simulink model "dyanmics_model"  (R2018b)
settings: Solver=VariableStepAuto  StartTime=0.0  StopTime=100.0  RelTol=1e-3
values from neighbouring files (symbols this model uses):
  aeroCoeff =     [flight_params.mat]
  alpha = [-15 -14 -13 -12 -11 -10 -9 -8 -7 -6 -5 -4 ... (31 elements, 1x31)]    [flight_params.mat]
  cjet = [0 1 2 3 4 5 6 7 8 9 10 11 ... (21 elements, 1x21)]    [flight_params.mat]
  CLtot = [-1.4145 -1.8537 -2.1722 -2.4757 -2.7723 -3.0649 -3.3548 -3.6428 -3.9294 -4.215 -4.4997 -4.7837 ... (13325 elements, 13x25x41)]    [flight_params.mat]
  CXtot = [0.3779 0.8471 1.6222 2.448 3.3002 4.1691 5.0501 5.94 6.8372 7.7403 8.6483 9.5605 ... (13325 elements, 13x25x41)]    [flight_params.mat]
  CZtot = [1.3677 1.6644 1.7212 1.7436 1.749 1.7441 1.732 1.7146 1.6931 1.6682 1.6407 1.6109 ... (13325 elements, 13x25x41)]    [flight_params.mat]
  environment =     [flight_params.mat]
  flap = [-10 -5 0 5 10 15 20 25 30 35 40 45 ... (21 elements, 1x21)]    [flight_params.mat]
  InitialConditions =     [flight_params.mat]
  vehicle =     [flight_params.mat]
libraries: simulink_extras x5, aerolibasang x2, shared3dof x1, sharedtransform x1
settings Model: Creator=Jacob  LastModifiedBy=Jacob

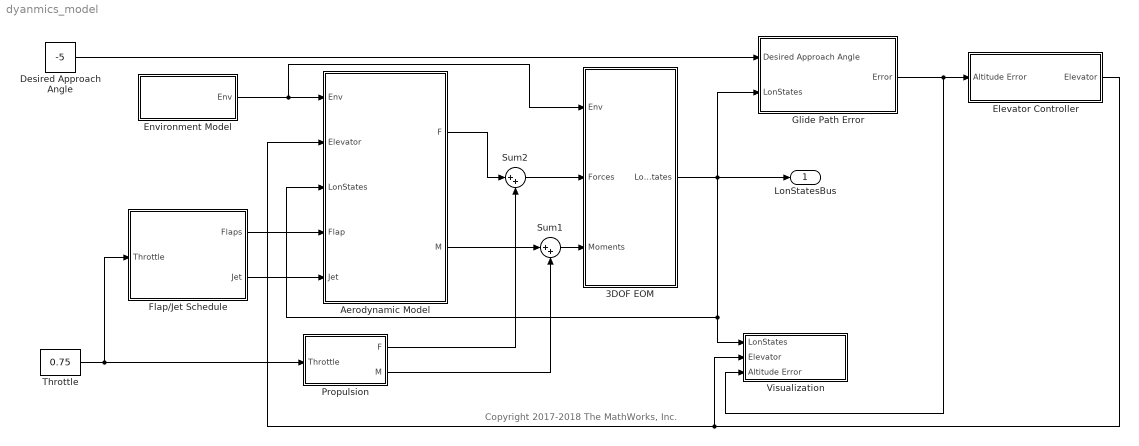
== system dyanmics_model ==
  note: Copyright 2017-2018 The MathWorks, Inc.
  3DOF EOM : Subsystem  VariantControl=eom3DOF
  Aerodynamic Model : Subsystem  VariantControl=aeroCONST
  Desired Approach Angle : Constant  Value=-5
  Elevator Controller : Subsystem
  Environment Model : Subsystem  mask(Constant Environment Model){To=environment.T0, a=environment.a, Po=environment.P0, AirDensity=environment.rho0, ugvgwg=environment.vel_wind, pgqgrg=environment.omega_wind, g=environment.grav}
      mask prompts: To "Constant Temperature (K):"; a "Constant Speed of Sound (m/s):"; Po "Constant Pressure (Pa):"; AirDensity "Constant Air Density (kg/m^3):"; ugvgwg "Constant Wind Velocity [ug vg wg] (m/s):"; pgqgrg "Constant Wind Angular Rates [pg qg rg] (rad/s):"; g "Constant Gravitational Acceleration (m/s^2):"
      mask Help: helpview(fullfile(docroot,'toolbox','aeroblks','aeroblks.map'), 'environment1');
      mask TypeOptions To: Constant Atmosphere/To
      mask TypeOptions a: Constant Atmosphere/a
      mask TypeOptions Po: Constant Atmosphere/Po
      mask TypeOptions AirDensity: Constant Atmosphere/AirDensity
      mask TypeOptions ugvgwg: Constant Wind/ugvgwg
      mask TypeOptions pgqgrg: Constant Wind/pgqgrg
      mask TypeOptions g: Constant Gravity/g
      mask DialogControl Container4 Prompt: Atmospheric Model
      mask DialogControl Container6 Prompt: Wind Model
      mask DialogControl Container8 Prompt: Gravity Model
      mask Display:
      | image('aeroenvironment.bmp','center')
      | port_label('output',1,'Env')
  Flap/Jet Schedule : Subsystem
  Glide Path Error : Subsystem
  Propulsion : Subsystem
      settings: RTWSystemCode=Inline
  Sum1 : Sum  Inputs=|++  SaturateOnIntegerOverflow=on  InputSameDT=on  OutDataTypeStr=Inherit: Same as first input
  Sum2 : Sum  Inputs=|++  SaturateOnIntegerOverflow=on  InputSameDT=on  OutDataTypeStr=Inherit: Same as first input
  Throttle : Constant  Value=0.75
  Visualization : Subsystem
  LonStatesBus : Outport
  wires:
  Propulsion/2(M) -> Sum1/2
  Propulsion/1(F) -> Sum2/2
  Environment Model/1(Env) -> 3DOF EOM/1(Env), Aerodynamic Model/1(Env)
  Sum1/1 -> 3DOF EOM/3(Moments)
  Aerodynamic Model/1(F) -> Sum2/1
  3DOF EOM/1(LonStates) -> Visualization/1(LonStates), Aerodynamic Model/3(LonStates), LonStatesBus/1, Glide Path Error/2(LonStates)
  Throttle/1 -> Flap/Jet Schedule/1(Throttle), Propulsion/1(Throttle)
  Sum2/1 -> 3DOF EOM/2(Forces)
  Aerodynamic Model/2(" M") -> Sum1/1
  Flap/Jet Schedule/2(Jet) -> Aerodynamic Model/5(Jet)
  Flap/Jet Schedule/1(Flaps) -> Aerodynamic Model/4(Flap)
  Desired Approach Angle/1 -> Glide Path Error/1(Desired Approach Angle)
  Glide Path Error/1(Error) -> Elevator Controller/1(Altitude Error), Visualization/3(Altitude Error)
  Elevator Controller/1(Elevator) -> Visualization/2(Elevator), Aerodynamic Model/2(Elevator)

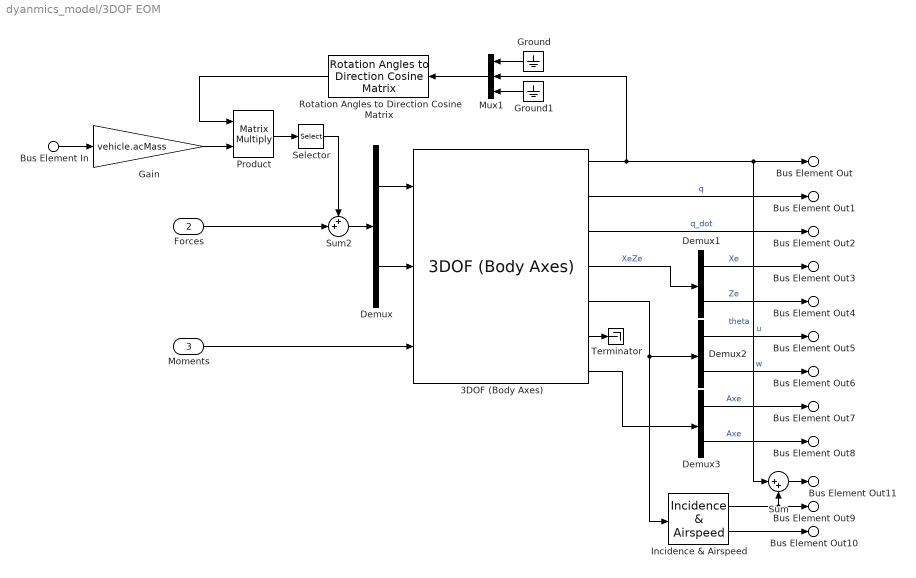
== system dyanmics_model/3DOF EOM ==
  Bus Element In : Inport  PortName=Env  Element=g
  Forces : Inport  Port=2
  Moments : Inport  Port=3
  3DOF (Body Axes) : shared3dof/3DOF (Body Axes)  units=Metric (MKS)  mtype=Fixed  v_ini=InitialConditions.v0  theta_ini=InitialConditions.theta0  alpha_ini=InitialConditions.alpha0  pos_ini=InitialConditions.x0  q_ini=InitialConditions.q0  mass=vehicle.acMass  mass_e=0.5  mass_f=3.0  Iyy=vehicle.inertia_yy  Iyy_e=0.5  Iyy_f=3.0  g_in=Internal  g=0  vre_flag=on  abi_flag=on  aMode=0  vel_statename={'u', 'w'}  theta_statename='theta'  pos_statename={'Xe', 'Ze'}  q_statename='q'  mass_statename=''
      settings: SourceProductName=Aerospace Blockset  SourceProductBaseCode=AE
  Demux{,1..3} (4 alike) : Demux  Outputs=2
  Gain : Gain  Gain=vehicle.acMass
  Ground : Ground
  Ground1 : Ground
  Incidence & Airspeed : aerolibasang/Incidence  & Airspeed
      settings: SourceProductName=Aerospace Blockset  SourceProductBaseCode=AE
  Mux1 : Mux  Inputs=3
  Product : Product  Multiplication=Matrix(*)
  Rotation Angles to Direction Cosine Matrix : sharedtransform/Rotation Angles to Direction Cosine Matrix  rotationOrder=ZYX  aMode=aMode
      settings: SourceProductBaseCode=AE
  Selector : Selector  InputPortWidth=3  IndexOptions=Index vector (dialog)  Indices=[1 3]  OutputSizes=1
  Sum : Sum  Inputs=|++
  Sum2 : Sum  Inputs=++|  SaturateOnIntegerOverflow=on  InputSameDT=on  OutDataTypeStr=Inherit: Same as first input
  Terminator : Terminator
  Bus Element Out : Outport  PortName=LonStates  Element=theta
  Bus Element Out1 : Outport  PortName=LonStates  Element=q
  Bus Element Out2 : Outport  PortName=LonStates  Element=q_dot
  Bus Element Out3 : Outport  PortName=LonStates  Element=Xe
  Bus Element Out4 : Outport  PortName=LonStates  Element=Ze
  Bus Element Out5 : Outport  PortName=LonStates  Element=u
  Bus Element Out6 : Outport  PortName=LonStates  Element=w
  Bus Element Out7 : Outport  PortName=LonStates  Element=Axe
  Bus Element Out8 : Outport  PortName=LonStates  Element=Aze
  Bus Element Out9 : Outport  PortName=LonStates  Element=alpha
  Bus Element Out10 : Outport  PortName=LonStates  Element=v
  Bus Element Out11 : Outport  PortName=LonStates  Element=gamma
  wires:
  Demux/2 -> 3DOF (Body Axes)/2
  Demux/1 -> 3DOF (Body Axes)/1
  Sum2/1 -> Demux/1
  Selector/1 -> Sum2/1
  Ground1/1 -> Mux1/3
  Ground/1 -> Mux1/1
  Mux1/1 -> Rotation Angles to Direction Cosine Matrix/1
  Gain/1 -> Product/2
  Rotation Angles to Direction Cosine Matrix/1 -> Product/1
  Product/1 -> Selector/1
  Forces/1 -> Sum2/2
  Bus Element In/1 -> Gain/1
  Moments/1 -> 3DOF (Body Axes)/3
  3DOF (Body Axes)/1 -> Mux1/2, Bus Element Out/1, Sum/1  "theta"
  3DOF (Body Axes)/2 -> Bus Element Out1/1  "q"
  3DOF (Body Axes)/3 -> Bus Element Out2/1  "q_dot"
  3DOF (Body Axes)/4 -> Demux1/1  "XeZe"
  3DOF (Body Axes)/5 -> Incidence & Airspeed/1, Demux2/1
  3DOF (Body Axes)/7 -> Demux3/1
  Demux3/1 -> Bus Element Out7/1  "Axe"
  Demux3/2 -> Bus Element Out8/1  "Axe"
  Demux2/2 -> Bus Element Out6/1  "w"
  Demux2/1 -> Bus Element Out5/1  "u"
  Demux1/2 -> Bus Element Out4/1  "Ze"
  Demux1/1 -> Bus Element Out3/1  "Xe"
  3DOF (Body Axes)/6 -> Terminator/1
  Incidence & Airspeed/1 -> Bus Element Out9/1, Sum/2
  Incidence & Airspeed/2 -> Bus Element Out10/1
  Sum/1 -> Bus Element Out11/1

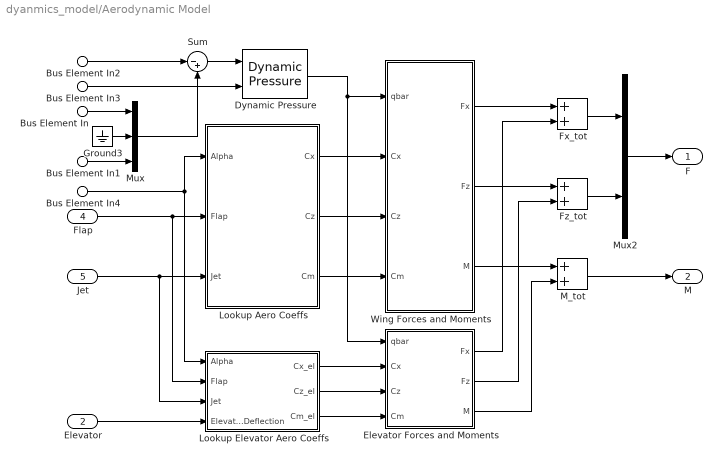
== system dyanmics_model/Aerodynamic Model ==
  Bus Element In2 : Inport  PortName=Env  Element=WindVelocity
  Bus Element In3 : Inport  PortName=Env  Element=AirDensity
  Elevator : Inport  Port=2
  Bus Element In : Inport  Port=3  PortName=LonStates  Element=u
  Bus Element In1 : Inport  Port=3  PortName=LonStates  Element=w
  Bus Element In4 : Inport  Port=3  PortName=LonStates  Element=alpha
  Flap : Inport  Port=4
  Jet : Inport  Port=5
  Dynamic Pressure : aerolibasang/Dynamic Pressure
  Elevator Forces and Moments : Subsystem
  Fx_tot : Sum  SaturateOnIntegerOverflow=on  InputSameDT=on  OutDataTypeStr=Inherit: Same as first input
  Fz_tot : Sum  SaturateOnIntegerOverflow=on  InputSameDT=on  OutDataTypeStr=Inherit: Same as first input
  Ground3 : Ground
  Lookup Aero Coeffs : Subsystem
  Lookup Elevator Aero Coeffs : Subsystem
  M_tot : Sum  SaturateOnIntegerOverflow=on  InputSameDT=on  OutDataTypeStr=Inherit: Same as first input
  Mux : Mux  Inputs=3
  Mux2 : Mux  Inputs=2
  Sum : Sum  Inputs=|-+
  Wing Forces and Moments : Subsystem
  F : Outport
  " M" : Outport  Port=2  Unit=N*m
  wires:
  Bus Element In3/1 -> Dynamic Pressure/2
  Bus Element In2/1 -> Sum/1
  Bus Element In/1 -> Mux/1
  Bus Element In1/1 -> Mux/3
  Mux2/1 -> F/1
  Ground3/1 -> Mux/2
  M_tot/1 -> " M"/1
  Sum/1 -> Dynamic Pressure/1
  Mux/1 -> Sum/2
  Elevator Forces and Moments/3(M) -> M_tot/2
  Dynamic Pressure/1 -> Elevator Forces and Moments/1(qbar), Wing Forces and Moments/1(qbar)
  Wing Forces and Moments/1(Fx) -> Fx_tot/1
  Wing Forces and Moments/3(M) -> M_tot/1
  Lookup Aero Coeffs/1(Cx) -> Wing Forces and Moments/2(Cx)
  Lookup Aero Coeffs/2(Cz) -> Wing Forces and Moments/3(Cz)
  Lookup Aero Coeffs/3(Cm) -> Wing Forces and Moments/4(Cm)
  Lookup Elevator Aero Coeffs/1(Cx_el) -> Elevator Forces and Moments/2(Cx)
  Lookup Elevator Aero Coeffs/2(Cz_el) -> Elevator Forces and Moments/3(Cz)
  Lookup Elevator Aero Coeffs/3(Cm_el) -> Elevator Forces and Moments/4(Cm)
  Elevator Forces and Moments/1(Fx) -> Fx_tot/2
  Elevator Forces and Moments/2(Fz) -> Fz_tot/2
  Wing Forces and Moments/2(Fz) -> Fz_tot/1
  Fx_tot/1 -> Mux2/1
  Fz_tot/1 -> Mux2/2
  Elevator/1 -> Lookup Elevator Aero Coeffs/4(Elevator Deflection)
  Flap/1 -> Lookup Elevator Aero Coeffs/2(Flap), Lookup Aero Coeffs/2(Flap)
  Jet/1 -> Lookup Elevator Aero Coeffs/3(Jet), Lookup Aero Coeffs/3(Jet)
  Bus Element In4/1 -> Lookup Elevator Aero Coeffs/1(Alpha), Lookup Aero Coeffs/1(Alpha)

== system dyanmics_model/Elevator Controller ==
  Altitude Error : Inport
  Gain : Gain  Gain=-0.00001  OutMin=vehicle.elevator_min/57.2958  OutMax=vehicle.elevator_max/57.2958
  Saturation : Saturate  UpperLimit=deg2rad(vehicle.elevator_max)  LowerLimit=deg2rad(vehicle.elevator_min)
  Elevator : Outport
  wires:
  Gain/1 -> Saturation/1
  Saturation/1 -> Elevator/1
  Altitude Error/1 -> Gain/1

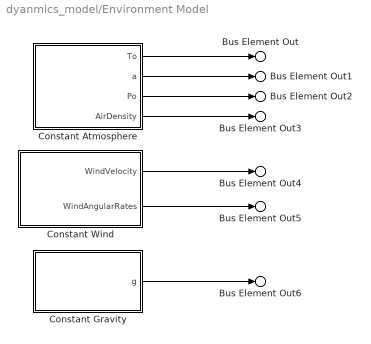
== system dyanmics_model/Environment Model ==
  Constant Atmosphere : Subsystem  VariantControl=atmosCONST  mask(Standard Atmospheric Constants){To=To, a=a, Po=Po, AirDensity=AirDensity}
      mask prompts: To "Constant Temperature (K):"; a "Constant Speed of Sound (m/s):"; Po "Constant Pressure (Pa):"; AirDensity "Constant Air Density (kg/m^3):"
  Constant Gravity : Subsystem  VariantControl=gravCONST  mask(Constant Gravitational Acceleration){g=g}
      mask prompts: g "Constant Gravitational Acceleration (m/s^2):"
  Constant Wind : Subsystem  VariantControl=windCONST  mask(Constant Wind Values){ugvgwg=ugvgwg, pgqgrg=pgqgrg}
      mask prompts: ugvgwg "Constant Wind Velocity (m/s):"; pgqgrg "Constant Wind Angular Rates (rad/s):"
  Bus Element Out : Outport  PortName=Env  Element=To
  Bus Element Out1 : Outport  PortName=Env  Element=a
  Bus Element Out2 : Outport  PortName=Env  Element=Po
  Bus Element Out3 : Outport  PortName=Env  Element=AirDensity
  Bus Element Out4 : Outport  PortName=Env  Element=WindVelocity
  Bus Element Out5 : Outport  PortName=Env  Element=WindAngularRates
  Bus Element Out6 : Outport  PortName=Env  Element=g
  wires:
  Constant Wind/2(WindAngularRates) -> Bus Element Out5/1
  Constant Atmosphere/3(Po) -> Bus Element Out2/1
  Constant Atmosphere/4(AirDensity) -> Bus Element Out3/1
  Constant Atmosphere/1(To) -> Bus Element Out/1
  Constant Wind/1(WindVelocity) -> Bus Element Out4/1
  Constant Atmosphere/2(a) -> Bus Element Out1/1
  Constant Gravity/1(g) -> Bus Element Out6/1

== system dyanmics_model/Flap//Jet Schedule ==
  Throttle : Inport
  Constant : Constant  Value=0
  Constant1 : Constant  Value=0
  Terminator : Terminator
  Flaps : Outport
  Jet : Outport  Port=2
  wires:
  Throttle/1 -> Terminator/1
  Constant/1 -> Jet/1
  Constant1/1 -> Flaps/1

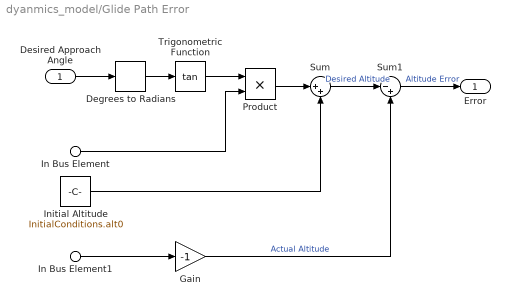
== system dyanmics_model/Glide Path Error ==
  Desired Approach Angle : Inport
  In Bus Element : Inport  Port=2  PortName=LonStates  Element=Xe
  In Bus Element1 : Inport  Port=2  PortName=LonStates  Element=Ze
  Degrees to Radians : simulink_extras/Transformations/Degrees to Radians
  Gain : Gain  Gain=-1
  "Initial Altitude " : Constant  Value=InitialConditions.alt0
  Product : Product
  Sum : Sum  Inputs=|++
  Sum1 : Sum  Inputs=|-+
  Trigonometric Function : Trigonometry  Operator=tan
  Error : Outport
  wires:
  Desired Approach Angle/1 -> Degrees to Radians/1
  Degrees to Radians/1 -> Trigonometric Function/1
  Trigonometric Function/1 -> Product/1
  In Bus Element/1 -> Product/2
  Product/1 -> Sum/1
  "Initial Altitude "/1 -> Sum/2
  In Bus Element1/1 -> Gain/1
  Sum/1 -> Sum1/1  "Desired Altitude"
  Sum1/1 -> Error/1  "Altitude Error"
  Gain/1 -> Sum1/2  "Actual Altitude"

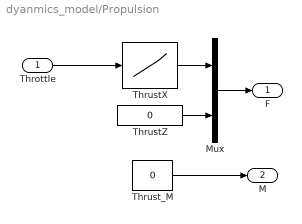
== system dyanmics_model/Propulsion ==
  Throttle : Inport
  Mux : Mux  Inputs=2
  ThrustX : Lookup_n-D  NumberOfTableDimensions=1  LookupTableObject=''  BreakpointsForDimension1=(1/6)*(3+([-3:3]))  IndexSearchMethod=Linear search  BeginIndexSearchUsingPreviousIndexResult=on  Table=vehicle.Thrust*(1+tanh([-3:3]))  ExtrapMethod=Clip  InputSameDT=on
  ThrustZ : Constant  Value=0  SampleTime=-1
  Thrust_M : Constant  Value=0  SampleTime=-1
  F : Outport  Unit=N
  M : Outport  Port=2  Unit=N*m
  wires:
  Throttle/1 -> ThrustX/1
  Thrust_M/1 -> M/1
  Mux/1 -> F/1
  ThrustZ/1 -> Mux/2
  ThrustX/1 -> Mux/1

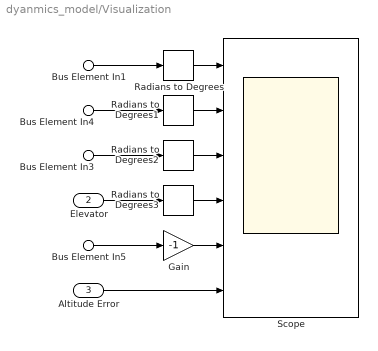
== system dyanmics_model/Visualization ==
  Bus Element In3 : Inport  PortName=LonStates  Element=gamma
  Bus Element In4 : Inport  PortName=LonStates  Element=theta
  Bus Element In5 : Inport  PortName=LonStates  Element=Ze
  Bus Element In1 : Inport  PortName=LonStates  Element=alpha
  Elevator : Inport  Port=2
  Altitude Error : Inport  Port=3
  Gain : Gain  Gain=-1
  Radians to Degrees{,1..3} (4 alike) : simulink_extras/Transformations/Radians to Degrees
  Scope : Scope  NumInputPorts=6
  wires:
  Bus Element In5/1 -> Gain/1
  Bus Element In3/1 -> Radians to Degrees2/1
  Radians to Degrees/1 -> Scope/1
  Bus Element In4/1 -> Radians to Degrees1/1
  Radians to Degrees1/1 -> Scope/2
  Elevator/1 -> Radians to Degrees3/1
  Gain/1 -> Scope/5
  Radians to Degrees3/1 -> Scope/4
  Bus Element In1/1 -> Radians to Degrees/1
  Radians to Degrees2/1 -> Scope/3
  Altitude Error/1 -> Scope/6

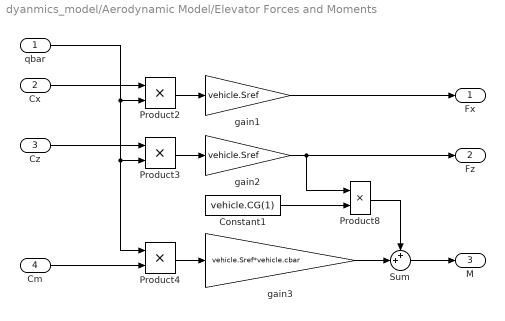
== system dyanmics_model/Aerodynamic Model/Elevator Forces and Moments ==
  qbar : Inport
  Cx : Inport  Port=2
  Cz : Inport  Port=3
  Cm : Inport  Port=4
  Constant1 : Constant  Value=vehicle.CG(1)
  Product2 : Product  SaturateOnIntegerOverflow=on  InputSameDT=on  OutDataTypeStr=Inherit: Same as first input
  Product3 : Product  SaturateOnIntegerOverflow=on  InputSameDT=on  OutDataTypeStr=Inherit: Same as first input
  Product4 : Product  SaturateOnIntegerOverflow=on  InputSameDT=on  OutDataTypeStr=Inherit: Same as first input
  Product8 : Product
  Sum : Sum  Inputs=++|
  gain1 : Gain  Gain=vehicle.Sref  SaturateOnIntegerOverflow=on  OutDataTypeStr=Inherit: Same as input  ParamDataTypeStr=Inherit: Same as input
  "gain2 " : Gain  Gain=vehicle.Sref  SaturateOnIntegerOverflow=on  OutDataTypeStr=Inherit: Same as input  ParamDataTypeStr=Inherit: Same as input
  gain3 : Gain  Gain=vehicle.Sref*vehicle.cbar  SaturateOnIntegerOverflow=on  OutDataTypeStr=Inherit: Same as input  ParamDataTypeStr=Inherit: Same as input
  Fx : Outport
  Fz : Outport  Port=2
  M : Outport  Port=3
  wires:
  Sum/1 -> M/1
  "gain2 "/1 -> Product8/1, Fz/1
  Constant1/1 -> Product8/2
  Product8/1 -> Sum/1
  gain3/1 -> Sum/2
  gain1/1 -> Fx/1
  Cx/1 -> Product2/1
  Cz/1 -> Product3/1
  Product3/1 -> "gain2 "/1
  Cm/1 -> Product4/2
  Product2/1 -> gain1/1
  Product4/1 -> gain3/1
  qbar/1 -> Product2/2, Product3/2, Product4/1

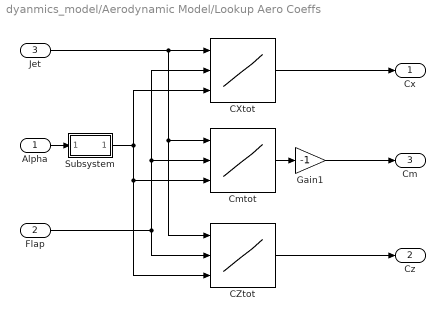
== system dyanmics_model/Aerodynamic Model/Lookup Aero Coeffs ==
  Alpha : Inport  Unit=rad
  Flap : Inport  Port=2  Unit=rad
  Jet : Inport  Port=3  Unit=rad
  CXtot : Lookup_n-D  NumberOfTableDimensions=3  BreakpointsForDimension1=cjet  BreakpointsForDimension2=flap  BreakpointsForDimension3=alpha  Table=CXtot  InternalRulePriority=Speed  RndMeth=Simplest  InputSameDT=on
  CZtot : Lookup_n-D  NumberOfTableDimensions=3  BreakpointsForDimension1=cjet  BreakpointsForDimension2=flap  BreakpointsForDimension3=alpha  Table=CZtot  InternalRulePriority=Speed  RndMeth=Simplest  InputSameDT=on
  Cmtot : Lookup_n-D  NumberOfTableDimensions=3  BreakpointsForDimension1=cjet  BreakpointsForDimension2=flap  BreakpointsForDimension3=alpha  Table=CLtot  InternalRulePriority=Speed  RndMeth=Simplest  InputSameDT=on
  Gain1 : Gain  Gain=-1
  Subsystem : Subsystem
      mask Display:
      | port_label('output',1,'deg')
      | port_label('input',1,'rad')
  Cx : Outport
  Cz : Outport  Port=2
  Cm : Outport  Port=3
  wires:
  Subsystem/1(Out2) -> CXtot/3, CZtot/3, Cmtot/3
  Alpha/1 -> Subsystem/1(In1)
  Flap/1 -> CXtot/2, Cmtot/2, CZtot/2
  Jet/1 -> CZtot/1, Cmtot/1, CXtot/1
  CXtot/1 -> Cx/1
  CZtot/1 -> Cz/1
  Cmtot/1 -> Gain1/1
  Gain1/1 -> Cm/1

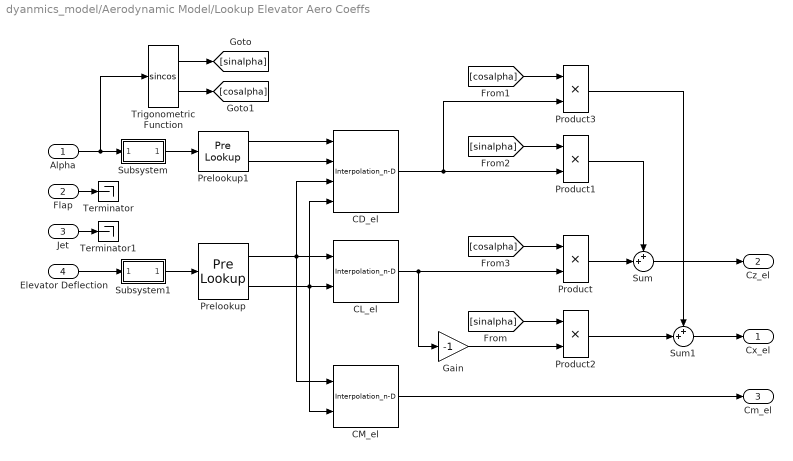
== system dyanmics_model/Aerodynamic Model/Lookup Elevator Aero Coeffs ==
  Alpha : Inport  Unit=rad
  Flap : Inport  Port=2  Unit=rad
  Jet : Inport  Port=3  Unit=rad
  Elevator Deflection : Inport  Port=4  Unit=rad
  CD_el : Interpolation_n-D  Table=aeroCoeff.CD_el
  CL_el : Interpolation_n-D  NumberOfTableDimensions=1  Table=aeroCoeff.CL_el  InternalRulePriority=Speed
      settings: InputPortMap=u0,u1
  CM_el : Interpolation_n-D  NumberOfTableDimensions=1  Table=aeroCoeff.CM_el  InternalRulePriority=Speed
      settings: InputPortMap=u0,u1
  Gain : Gain  Gain=-1
  Prelookup : PreLookup  BreakpointsData=aeroCoeff.def_vec  ExtrapMethod=Linear  IndexDataTypeStr=int32  FractionDataTypeStr=double
  Prelookup1 : PreLookup  BreakpointsData=aeroCoeff.alpha_vec  ExtrapMethod=Linear  IndexDataTypeStr=int32  FractionDataTypeStr=double
  Product{,1..3} (4 alike) : Product
  Subsystem : Subsystem
      mask Display:
      | port_label('output',1,'deg')
      | port_label('input',1,'rad')
  Subsystem1 : Subsystem
      mask Display:
      | port_label('output',1,'deg')
      | port_label('input',1,'rad')
  Sum : Sum  Inputs=++|
  Sum1 : Sum  Inputs=++|
  Terminator : Terminator
  Terminator1 : Terminator
  Trigonometric Function : Trigonometry  Operator=sincos
  Cx_el : Outport
  Cz_el : Outport  Port=2
  Cm_el : Outport  Port=3
  wires:
  Subsystem1/1(Out2) -> Prelookup/1
  Trigonometric Function/1 -> [sinalpha]
  Trigonometric Function/2 -> [cosalpha]
  [cosalpha] -> Product/1
  [cosalpha] -> Product3/1
  [sinalpha] -> Product1/1
  [sinalpha] -> Product2/1
  Prelookup1/2 -> CD_el/2
  Prelookup1/1 -> CD_el/1
  Elevator Deflection/1 -> Subsystem1/1(In1)
  Subsystem/1(Out2) -> Prelookup1/1
  Alpha/1 -> Trigonometric Function/1, Subsystem/1(In1)
  Prelookup/2 -> CM_el/2, CL_el/2, CD_el/4
  Prelookup/1 -> CD_el/3, CL_el/1, CM_el/1
  CD_el/1 -> Product3/2, Product1/2
  Gain/1 -> Product2/2
  Product3/1 -> Sum1/1
  CL_el/1 -> Gain/1, Product/2
  Product2/1 -> Sum1/2
  Product/1 -> Sum/2
  Product1/1 -> Sum/1
  Sum/1 -> Cz_el/1
  CM_el/1 -> Cm_el/1
  Sum1/1 -> Cx_el/1
  Flap/1 -> Terminator/1
  Jet/1 -> Terminator1/1

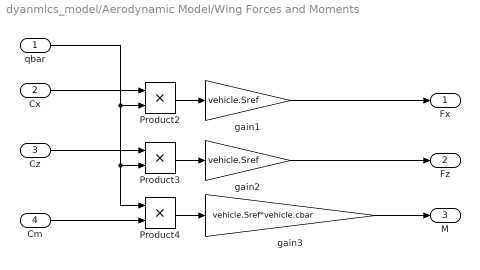
== system dyanmics_model/Aerodynamic Model/Wing Forces and Moments ==
  qbar : Inport
  Cx : Inport  Port=2
  Cz : Inport  Port=3
  Cm : Inport  Port=4
  Product2 : Product  SaturateOnIntegerOverflow=on  InputSameDT=on  OutDataTypeStr=Inherit: Same as first input
  Product3 : Product  SaturateOnIntegerOverflow=on  InputSameDT=on  OutDataTypeStr=Inherit: Same as first input
  Product4 : Product  SaturateOnIntegerOverflow=on  InputSameDT=on  OutDataTypeStr=Inherit: Same as first input
  gain1 : Gain  Gain=vehicle.Sref  SaturateOnIntegerOverflow=on  OutDataTypeStr=Inherit: Same as input  ParamDataTypeStr=Inherit: Same as input
  "gain2 " : Gain  Gain=vehicle.Sref  SaturateOnIntegerOverflow=on  OutDataTypeStr=Inherit: Same as input  ParamDataTypeStr=Inherit: Same as input
  gain3 : Gain  Gain=vehicle.Sref*vehicle.cbar  SaturateOnIntegerOverflow=on  OutDataTypeStr=Inherit: Same as input  ParamDataTypeStr=Inherit: Same as input
  Fx : Outport
  Fz : Outport  Port=2
  M : Outport  Port=3
  wires:
  gain3/1 -> M/1
  "gain2 "/1 -> Fz/1
  qbar/1 -> Product2/2, Product4/1, Product3/2
  Product4/1 -> gain3/1
  Product2/1 -> gain1/1
  Cm/1 -> Product4/2
  Product3/1 -> "gain2 "/1
  Cz/1 -> Product3/1
  Cx/1 -> Product2/1
  gain1/1 -> Fx/1

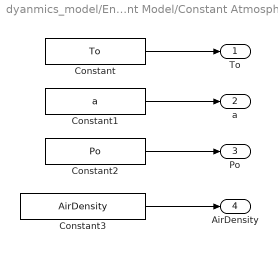
== system dyanmics_model/Environment Model/Constant Atmosphere ==
  Constant : Constant  Value=To
  Constant1 : Constant  Value=a
  Constant2 : Constant  Value=Po
  Constant3 : Constant  Value=AirDensity
  To : Outport
  a : Outport  Port=2
  Po : Outport  Port=3
  AirDensity : Outport  Port=4
  wires:
  Constant1/1 -> a/1
  Constant/1 -> To/1
  Constant2/1 -> Po/1
  Constant3/1 -> AirDensity/1

== system dyanmics_model/Environment Model/Constant Gravity ==
  Reshape1 : Reshape  OutputDimensionality=Column vector (2-D)
  Standard Gravity : Constant  Value=g
  g : Outport
  wires:
  Reshape1/1 -> g/1
  Standard Gravity/1 -> Reshape1/1

== system dyanmics_model/Environment Model/Constant Wind ==
  Reshape : Reshape  OutputDimensionality=Column vector (2-D)
  Reshape1 : Reshape  OutputDimensionality=Column vector (2-D)
  pg,qg,rg : Constant  Value=pgqgrg
  ug,vg,wg : Constant  Value=ugvgwg
  WindVelocity : Outport
  WindAngularRates : Outport  Port=2
  wires:
  pg,qg,rg/1 -> Reshape1/1
  ug,vg,wg/1 -> Reshape/1
  Reshape/1 -> WindVelocity/1
  Reshape1/1 -> WindAngularRates/1

== system dyanmics_model/Aerodynamic Model/Lookup Aero Coeffs/Subsystem ==
  In1 : Inport
  Signal Specification : SignalSpecification  Unit=deg
  Unit Conversion : UnitConversion
  Out2 : Outport
  wires:
  In1/1 -> Unit Conversion/1
  Unit Conversion/1 -> Signal Specification/1
  Signal Specification/1 -> Out2/1

== system dyanmics_model/Aerodynamic Model/Lookup Elevator Aero Coeffs/Subsystem ==
  In1 : Inport
  Signal Specification : SignalSpecification  Unit=deg
  Unit Conversion : UnitConversion
  Out2 : Outport
  wires:
  In1/1 -> Unit Conversion/1
  Unit Conversion/1 -> Signal Specification/1
  Signal Specification/1 -> Out2/1

== system dyanmics_model/Aerodynamic Model/Lookup Elevator Aero Coeffs/Subsystem1 ==
  In1 : Inport
  Signal Specification : SignalSpecification  Unit=deg
  Unit Conversion : UnitConversion
  Out2 : Outport
  wires:
  Signal Specification/1 -> Out2/1
  Unit Conversion/1 -> Signal Specification/1
  In1/1 -> Unit Conversion/1
